simulink model "AFCSModel"  (R2025b)
settings: Solver=ode4  StartTime=0.0  StopTime=200  FixedStep=0.01  RelTol=1e-3  EnableMultiTasking=on
values from neighbouring files (symbols this model uses):
  AD = [0.05526	0.05526	0.05568	0.05804	0.06460	0.08210 ... (first row only)    [AirCraftData.m]
  Alpha0 = [0.143	0.143	0.122	-0.267	-0.627	0.120 ... (first row only)    [AirCraftData.m]
  alt = 1284.73    [Start.m]    (also in drl_simplified_dynamics.m)
  CA = 3.451    [AirCraftData.m]    (also in AircraftTrim.m)
  CDmin = [0.03799	0.03799	0.03799	0.03799	0.03904	0.04277 ... (first row only)    [AirCraftData.m]
  CLAlpha = [0.1012	0.1021	0.1033	0.1051	0.1079	0.0976 ... (first row only)    [AirCraftData.m]
  Clbt0 = [-0.00147	-0.00148	-0.00149	-0.00153	-0.00158	-0.00171 ... (first row only)    [AirCraftData.m]
  Clbtaf = [0	0	0	0	0	0;0	 0	0	0	0	0]    [AirCraftData.m]
  ClDelA = [-0.003110	-0.003065	-0.003040	-0.003036	-0.003052	-0.003088 ... (first row only)    [AirCraftData.m]
  CLDelE = [0.00653	0.00668	0.00690	0.00724	0.00772	0.00846 ... (first row only)    [AirCraftData.m]
  ClDelR = [0.000584	0.000605	0.000638	0.000686	0.000760	0.000877 ... (first row only)    [AirCraftData.m]
  CLDM = [0.244	0.244	0.244	0.244	0.244	0.244 ... (first row only)    [AirCraftData.m]
  Clp0 = [-0.5510 	-0.5610 	-0.5767 	-0.6005 	-0.6224 	-0.6763 ... (first row only)    [AirCraftData.m]
  ClpAf = [0,0,0,0,0,0;0,0,0,0,0,0]    [AirCraftData.m]
  Clr0 = [0.1308 	0.1339 	0.1383 	0.1474 	0.1601 	0.1738 ... (first row only)    [AirCraftData.m]
  ClrAf = [0,0,0,0,0,0;0,0,0,0,0,0]    [AirCraftData.m]
  Cm0 = [0.2014	0.2017	0.2034	0.2083	0.2207	0.2475 ... (first row only)    [AirCraftData.m]
  CmAfdot = [-11.5890 	-12.0169 	-12.7558 	-13.8010 	-15.2088 	-16.2278 ... (first row only)    [AirCraftData.m]
  CmCl = [-0.3454	-0.3441	-0.3427	-0.3412	-0.3396	-0.3379 ... (first row only)    [AirCraftData.m]
  CmDelE = [-0.03554	-0.03651	-0.03802	-0.04028	-0.04365	-0.04798 ... (first row only)    [AirCraftData.m]
  Cmq0 = [-42.0260 	-42.2665 	-42.9499 	-44.8315 	-45.5877 	-46.0842 ... (first row only)    [AirCraftData.m]
  CN1A0 = [0.0740	0.0662	0.0605	0.0552	0.0554 ... (first row only)    [AirCraftData.m]
  Cnbt0 = [0.00180	0.00183	0.00187	0.00192	0.00200	0.00207 ... (first row only)    [AirCraftData.m]
  Cnbtaf = [-0.000030 	-0.000031 	-0.000031 	-0.000032 	-0.000033 	-0.000035 ... (first row only)    [AirCraftData.m]
  CnDelA0 = [-0.000180	-0.000178	-0.000176	-0.000176	-0.000177	-0.000179 ... (first row only)    [AirCraftData.m]
  CnDelAAf = [0	 0	0	0	0	0;0	 0	0	0	0	0]    [AirCraftData.m]
  CnDelR = [-0.002214	-0.002274	-0.002367	-0.002505	-0.002712	-0.003039 ... (first row only)    [AirCraftData.m]
  Cnp0 = [0.0521 	0.0532 	0.0571 	0.0601 	0.0636 	0.0664 ... (first row only)    [AirCraftData.m]
  CnpAf = [0,0,0,0,0,0;0,0,0,0,0,0]    [AirCraftData.m]
  Cnr = [-0.1810 	-0.1832 	-0.1855 	-0.1892 	-0.1933 	-0.1973 ... (first row only)    [AirCraftData.m]
  Cxh_Slip = [0.0000, 0.0045, 0.0089, 0.0132, 0.0174 ... (first row only)    [AirCraftData.m]
  Cybeta0 = [-0.01783	-0.01790	-0.01804	-0.01824	-0.01851	-0.01884 ... (first row only)    [AirCraftData.m]
  Cybtaf = [0 0 0 0 0 0;0 0 0 0 0 0]    [AirCraftData.m]
  CyDelA = [0.000287	0.000295	0.000307	0.000325	0.000351	0.000394 ... (first row only)    [AirCraftData.m]
  CyDelR = [0.004946	0.005035	0.005316	0.005791	0.006458	0.007318 ... (first row only)    [AirCraftData.m]
  Cyh_Slip = [0.0000, -0.0248, -0.0519, -0.0813, -0.1130 ... (first row only)    [AirCraftData.m]
  ETA_data = [0.729 0.727 0.72 0.71 0.877 0.858 0.855 0.853 0.857 0.862 0.87 0.796 ... (330 elements, 11x5x6)]    [ETA_data.mat]
  eul_0 = [0/57.3 0/57.3 0/57.3]    [AircraftTrim.m]
  F = A(:, 1)    [drl_simplified_dynamics.m]    (also in func_DrawAircraftModel.m = [         1,  2,  3,  1;         1,  3,  4,  1;         1,  )
  flap = 0    [AircraftTrim.m]
  inertia = [  Ix      Iy     Iz  Ixz]    [AircraftTrim.m]
  Initi_Heading = 15.95*pi/180    (= 0.278380015693)    [Start.m]
  Initi_Lati = 32.6261    [Start.m]
  Initi_Longi = 103.5940    (= 103.594)    [Start.m]
  mass = 54000    [Start.m]    (also in drl_simplified_dynamics.m)
  op = evalin('base', 'op')    [drl_simplified_dynamics.m]
  q = func_GreatCircleForward(start_lat, start_lon, leg_bearing, local_s)    [system_model_update.m]
  r = r1 + r2    [drl_piecewise_reward.m]    (also in drl_reward_function.m)
  RNPAR_FlightPlan = JiuZhaiHuangLong_RNPAR_FlightPlan    [Manuscript_RNPAR_FlightPlan.m]
  Vab_0 = [Vt 0 0]    [AircraftTrim.m]
  Vt = 80    [Start.m]    (also in drl_simplified_dynamics.m; setup_afcs_system_model_test.m)
  wind_direction = 0    [Start.m]
  wind_type = 2    [Start.m]
  Wxyz_0 = [0 0 0]    [AircraftTrim.m]
  X = 1.06    [AircraftTrim.m]
  xme_0 = [0 0 -alt]    [AircraftTrim.m]
  Y = 1.177    [AircraftTrim.m]
undefined symbols (not defined in the file or in its folder): func_SystemModelMonitorBlock, Light, MIL, slselsubs, thrust_data
libraries: simulink_extras x4, aerolibatmos2 x3, aerolibconvert2 x3, aerolibwind2 x3, sharedutil x2, aerolibobsolete x1
(part 1 of 3)
settings Model: Creator=Administrator  LastModifiedBy=19894
settings SolverCC: AlgebraicLoopSolver=TrustRegion
settings DataIOCC: LimitDataPoints=on  SaveFormat=Array  SignalLoggingSaveFormat=ModelDataLogs  ReturnWorkspaceOutputs=off
settings OptimizationCC: DefaultParameterBehavior=Inlined  BufferReuse=off  ExpressionDepthLimit=2147483647.0  InitFltsAndDblsToZero=on  LifeSpan=inf
settings DebuggingCC: AlgebraicLoopMsg=none  SaveWithParameterizedLinksMsg=none  UnderspecifiedInitializationDetection=Classic  MergeDetectMultiDrivingBlocksExec=none  SignalResolutionControl=TryResolveAllWithWarning  MultiTaskDSMMsg=warning  MultiTaskCondExecSysMsg=none  FcnCallInpInsideContextMsg=warning  StateNameClashWarn=warning  SFUnexpectedBacktrackingDiag=warning  SFNoUnconditionalDefaultTransitionDiag=warning  SFExecutionAtInitializationDiag=none  ArithmeticOperatorsInVariantConditions=warning
settings HardwareCC: ProdBitPerPointer=32.0  ProdBitPerSizeT=32.0  ProdBitPerPtrDiffT=32.0  ProdLargestAtomicFloat=None  ProdIntDivRoundTo=Undefined  ProdEndianess=Unspecified  ProdWordSize=32.0  ProdHWDeviceType=32-bit Generic
settings ModelReferenceCC: PropagateSignalLabelsOutOfModel=off
settings SFSimCC: SimUseLocalCustomCode=off  CustomCodeUndefinedFunction=UseInterfaceOnly
settings RTWCC: RTWUseLocalCustomCode=off  GPUComputeCapability=3.5
settings CodeAppCC: StateflowObjectComments=on
settings GRTTargetCC: TargetFcnLib=ansi_tfl_tmw.mat  TargetLangStandard=C89/C90 (ANSI)  CombineOutputUpdateFcns=off  GRTInterface=on
settings ConfigComp: CovMetricSettings=dw  CovSaveCumulativeToWorkspaceVar=on  CovSaveSingleToWorkspaceVar=on  CovExternalEMLEnable=off  CovSFcnEnable=off

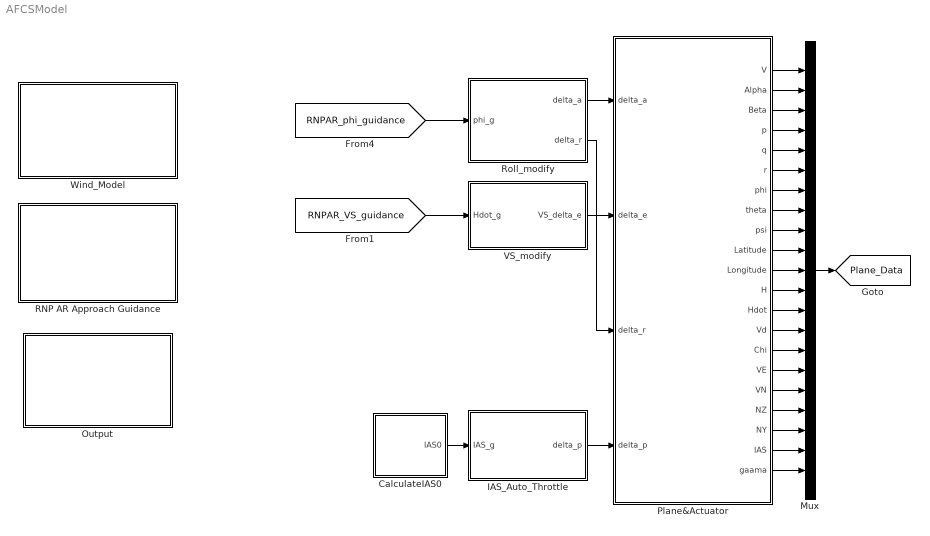
== system AFCSModel ==
  CalculateIAS0 : Subsystem
  IAS_Auto_Throttle : Subsystem
  Mux : Mux  Inputs=21
  Output : Subsystem
  Plane&Actuator : Subsystem
  RNP AR Approach Guidance : Subsystem
  Roll_modify : Subsystem
  VS_modify : Subsystem
  Wind_Model : Subsystem
  tag scope: Plane_Data=global
  wires:
  Plane&Actuator/3(Beta) -> Mux/3
  Plane&Actuator/2(Alpha) -> Mux/2
  Plane&Actuator/5(q) -> Mux/5
  Plane&Actuator/4(p) -> Mux/4
  Plane&Actuator/1(V) -> Mux/1
  Plane&Actuator/10(Latitude) -> Mux/10
  Plane&Actuator/7(phi) -> Mux/7
  Plane&Actuator/9(psi) -> Mux/9
  Plane&Actuator/12(H) -> Mux/12
  Plane&Actuator/6(r) -> Mux/6
  Plane&Actuator/11(Longitude) -> Mux/11
  Plane&Actuator/13(Hdot) -> Mux/13
  Plane&Actuator/17(VN) -> Mux/17
  Plane&Actuator/18(NZ) -> Mux/18
  Plane&Actuator/20(IAS) -> Mux/20
  Plane&Actuator/15(Chi) -> Mux/15
  Plane&Actuator/16(VE) -> Mux/16
  Plane&Actuator/19(NY) -> Mux/19
  Plane&Actuator/14(Vd) -> Mux/14
  Plane&Actuator/8(theta) -> Mux/8
  Mux/1 -> [Plane_Data]
  Plane&Actuator/21(gaama) -> Mux/21
  VS_modify/1(VS_delta_e) -> Plane&Actuator/2(delta_e)
  Roll_modify/1(delta_a) -> Plane&Actuator/1(delta_a)
  Roll_modify/2(delta_r) -> Plane&Actuator/3(delta_r)
  IAS_Auto_Throttle/1(delta_p) -> Plane&Actuator/4(delta_p)
  CalculateIAS0/1(IAS0) -> IAS_Auto_Throttle/1(IAS_g)
  [RNPAR_VS_guidance] -> VS_modify/1(Hdot_g)
  [RNPAR_phi_guidance] -> Roll_modify/1(phi_g)

== system AFCSModel/CalculateIAS0 ==
  Constant : Constant  Value=Vt
  Constant1 : Constant  Value=alt
  TAS-EAS1 : Subsystem
  IAS0 : Outport
  wires:
  Constant/1 -> TAS-EAS1/1(TAS  (m/s))
  Constant1/1 -> TAS-EAS1/2(Height  (m))
  TAS-EAS1/1(EAS (m/s)) -> IAS0/1

== system AFCSModel/IAS_Auto_Throttle ==
  IAS_g : Inport
  IAS_Controller : Subsystem
  Selector2 : Selector  InputPortWidth=21  IndexOptions=Index vector (dialog)  Indices=20  OutputSizes=1
  delta_p : Outport
  wires:
  IAS_g/1 -> IAS_Controller/1(IAS_g)
  IAS_Controller/1(delta_p) -> delta_p/1
  [Plane_Data] -> Selector2/1
  Selector2/1 -> IAS_Controller/2(IAS)

== system AFCSModel/Output ==
  note: Plane_Data  Unit:
      | V:                    m/s
      | Alpha:             rad
      | Beta:               rad
      | p:                    rad/s
      | q:                    rad/s
      | r:                     rad/s
      | phi:                 rad
      | theta:              rad
      | psi:                  rad
      | Latitude:         deg
      | Longitude:      deg
      | H:                    m
      | Hdot:               m/s
      | Vd:                  m/s
      | Chi:                 rad
      | VE:                  m/s
      | VN:                  m/s
      | NZ:                    \
      | NY:                    \
      | IAS:                 m/s
      | gaama：         rad
  Clock : Clock
  Constant : Constant  Value=110
  Gain : Gain  Gain=180/pi
  Integrator : Integrator
  Relational Operator : RelationalOperator  Operator=<=  OutDataTypeStr=boolean  InputSameDT=off
  Scope : Scope
  Scope1 : Scope
      settings: DataLoggingVariableName=ScopeData3
  Selector1 : Selector  InputPortWidth=21  IndexOptions=Index vector (dialog)  Indices=1  OutputSizes=1
  Selector2 : Selector  InputPortWidth=21  IndexOptions=Index vector (dialog)  Indices=10  OutputSizes=1
  Selector3 : Selector  InputPortWidth=21  IndexOptions=Index vector (dialog)  Indices=11  OutputSizes=1
  Selector4 : Selector  InputPortWidth=21  IndexOptions=Index vector (dialog)  Indices=12  OutputSizes=1
  Selector5 : Selector  InputPortWidth=21  IndexOptions=Index vector (dialog)  Indices=14  OutputSizes=1
  Selector6 : Selector  InputPortWidth=21  IndexOptions=Index vector (dialog)  Indices=20  OutputSizes=1
  Selector7 : Selector  InputPortWidth=21  IndexOptions=Index vector (dialog)  Indices=9  OutputSizes=1
  Stop Simulation : Stop
  To Workspace1 : ToWorkspace  VariableName=Plane_TAS  SampleTime=-1
  To Workspace2 : ToWorkspace  VariableName=Plane_Lati  SampleTime=-1
  To Workspace3 : ToWorkspace  VariableName=Plane_Longi  SampleTime=-1
  To Workspace4 : ToWorkspace  VariableName=Plane_Height  SampleTime=-1
  To Workspace5 : ToWorkspace  VariableName=Plane_Vground  SampleTime=-1
  To Workspace6 : ToWorkspace  VariableName=Plane_IAS  SampleTime=-1
  To Workspace7 : ToWorkspace  VariableName=Sim_time  SampleTime=-1
  To Workspace8 : ToWorkspace  VariableName=FlightDistance  SampleTime=-1
  wires:
  [Plane_Data] -> Selector7/1, Selector6/1, Selector5/1, Selector4/1, Selector2/1, Selector3/1, Selector1/1
  Selector1/1 -> To Workspace1/1
  Selector2/1 -> To Workspace2/1
  Selector3/1 -> To Workspace3/1
  Selector4/1 -> Relational Operator/1, Scope/1, To Workspace4/1
  Selector5/1 -> Integrator/1, To Workspace5/1
  Selector6/1 -> To Workspace6/1
  Selector7/1 -> Gain/1
  Gain/1 -> Scope1/1
  Clock/1 -> To Workspace7/1
  Relational Operator/1 -> Stop Simulation/1
  Constant/1 -> Relational Operator/2
  Integrator/1 -> To Workspace8/1

== system AFCSModel/Plane&Actuator ==
  note: Plane_Data  Unit:
      | V:                    m/s
      | Alpha:             rad
      | Beta:               rad
      | p:                    rad/s
      | q:                    rad/s
      | r:                     rad/s
      | phi:                 rad
      | theta:              rad
      | psi:                  rad
      | Latitude:         deg
      | Longitude:      deg
      | H:                    m
      | Hdot:               m/s
      | Vd:                  m/s
      | Chi:                 rad
      | VE:                  m/s
      | VN:                  m/s
      | NZ:                    \
      | NY:                    \
      | IAS:                 m/s
      | gaama：         rad
  delta_a : Inport
  delta_e : Inport  Port=2
  delta_r : Inport  Port=3
  delta_p : Inport  Port=4
  Actuator : Subsystem
  PlaneModel : Subsystem
  V : Outport
  Alpha : Outport  Port=2
  Beta : Outport  Port=3
  p : Outport  Port=4
  q : Outport  Port=5
  r : Outport  Port=6
  phi : Outport  Port=7
  theta : Outport  Port=8
  psi : Outport  Port=9
  Latitude : Outport  Port=10
  Longitude : Outport  Port=11
  H : Outport  Port=12
  Hdot : Outport  Port=13
  Vd : Outport  Port=14
  Chi : Outport  Port=15
  VE : Outport  Port=16
  VN : Outport  Port=17
  NZ : Outport  Port=18
  NY : Outport  Port=19
  IAS : Outport  Port=20
  gaama : Outport  Port=21
  wires:
  delta_a/1 -> Actuator/1(delta_a_c)
  delta_e/1 -> Actuator/2(delta_e_c)
  delta_r/1 -> Actuator/3(delta_r_c)
  delta_p/1 -> Actuator/4(delta_p_c)
  PlaneModel/1(V) -> V/1
  PlaneModel/2(Alpha) -> Alpha/1
  PlaneModel/3(Beta) -> Beta/1
  PlaneModel/4(p) -> p/1
  PlaneModel/5(q) -> q/1
  PlaneModel/6(r) -> r/1
  PlaneModel/7(phi) -> phi/1
  PlaneModel/9(psi) -> psi/1
  PlaneModel/10(Latitude) -> Latitude/1
  PlaneModel/11(Longitude) -> Longitude/1
  PlaneModel/12(H) -> H/1
  PlaneModel/13(Hdot) -> Hdot/1
  PlaneModel/14(Vd) -> Vd/1
  PlaneModel/15(Chi) -> Chi/1
  PlaneModel/16(VE) -> VE/1
  PlaneModel/17(VN) -> VN/1
  PlaneModel/18(NZ) -> NZ/1
  PlaneModel/19(NY) -> NY/1
  PlaneModel/20(IAS) -> IAS/1
  PlaneModel/21(gaama) -> gaama/1
  PlaneModel/8(theta) -> theta/1
  Actuator/1(delta_a) -> PlaneModel/1(delta_a)
  Actuator/2(delta_e) -> PlaneModel/2(delta_e)
  Actuator/3(delta_r) -> PlaneModel/3(delta_r)
  Actuator/4(delta_p) -> PlaneModel/4(delta_p)

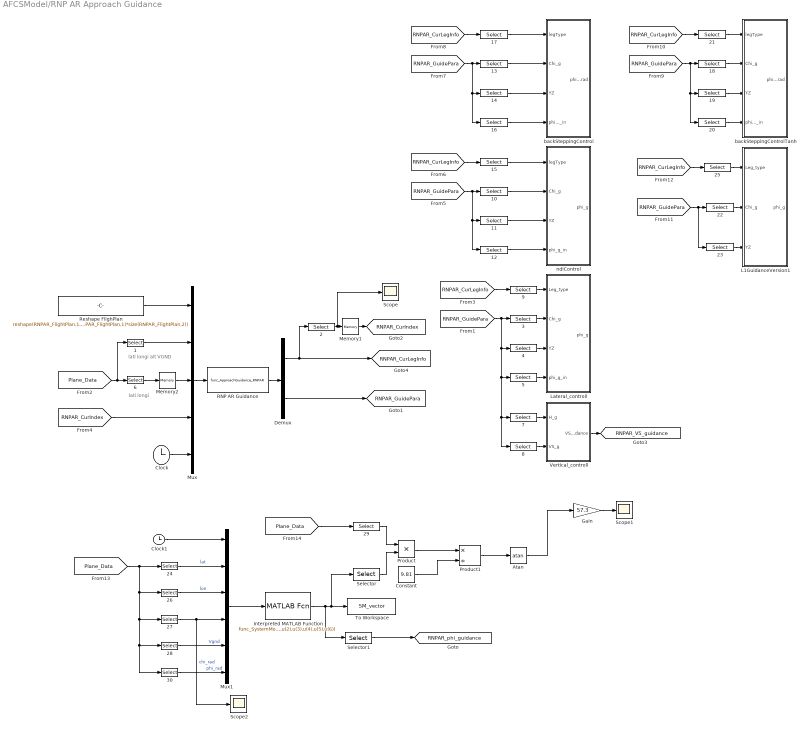
== system AFCSModel/RNP AR Approach Guidance ==
  note: lati
      | longi
  note: lati
      | longi
      | alt
      | VGND
  1 : Selector  InputPortWidth=21  IndexOptions=Index vector (dialog)  Indices=[10 11 12 14]  OutputSizes=[(-2)]
  {3,10,13,18,22} (5 alike) : Selector  InputPortWidth=5  IndexOptions=Index vector (dialog)  Indices=2  OutputSizes=[(-2)]
  {4,11,14,19,23} (5 alike) : Selector  InputPortWidth=5  IndexOptions=Index vector (dialog)  Indices=1  OutputSizes=[(-2)]
  {5,12,16,20} (4 alike) : Selector  InputPortWidth=5  IndexOptions=Index vector (dialog)  Indices=3  OutputSizes=[(-2)]
  {9,15,17,21,25} (5 alike) : Selector  InputPortWidth=16  IndexOptions=Index vector (dialog)  Indices=4  OutputSizes=[(-2)]
  2 : Selector  InputPortWidth=16  IndexOptions=Index vector (dialog)  Indices=2  OutputSizes=[(-2)]
  24 : Selector  InputPortWidth=21  IndexOptions=Index vector (dialog)  Indices=10  OutputSizes=[(-2)]
  26 : Selector  InputPortWidth=21  IndexOptions=Index vector (dialog)  Indices=11  OutputSizes=[(-2)]
  27 : Selector  InputPortWidth=21  IndexOptions=Index vector (dialog)  Indices=15  OutputSizes=[(-2)]
  28 : Selector  InputPortWidth=21  IndexOptions=Index vector (dialog)  Indices=14  OutputSizes=[(-2)]
  29 : Selector  InputPortWidth=21  IndexOptions=Index vector (dialog)  Indices=14  OutputSizes=[(-2)]
  30 : Selector  InputPortWidth=21  IndexOptions=Index vector (dialog)  Indices=7  OutputSizes=[(-2)]
  6 : Selector  InputPortWidth=21  IndexOptions=Index vector (dialog)  Indices=[10 11]  OutputSizes=[(-2)]
  7 : Selector  InputPortWidth=5  IndexOptions=Index vector (dialog)  Indices=4  OutputSizes=[(-2)]
  8 : Selector  InputPortWidth=5  IndexOptions=Index vector (dialog)  Indices=5  OutputSizes=[(-2)]
  Atan : Trigonometry  Operator=atan
  Clock : Clock
  Clock1 : Clock
  Constant : Constant  Value=9.81
  Demux : Demux  Outputs=[16 5]
  Gain : Gain  Gain=57.3
  Interpreted MATLAB Function : MATLABFcn  MATLABFcn=func_SystemModelMonitorBlock(u(1),u(2),u(3),u(4),u(5),u(6))  OutputDimensions=14
  L1GuidanceVersion1 : Subsystem
  Lateral_controll : Subsystem
  Memory1 : Memory  InitialCondition=1
  Memory2 : Memory  InitialCondition=1
  Mux : Mux  Inputs=5
  Mux1 : Mux  Inputs=6
  Product : Product
  Product1 : Product  Inputs=*/
  RNP AR Guidance : MATLABFcn  MATLABFcn=func_ApproachGuidance_RNPAR  OutputDimensions=21
  Reshape FlighPlan : Constant  Value=reshape(RNPAR_FlightPlan,1,size(RNPAR_FlightPlan,1)*size(RNPAR_FlightPlan,2))
  Scope : Scope
      settings: ActiveDisplayYMinimum=-1  ActiveDisplayYMaximum=1  DataLoggingVariableName=ScopeData2
  Scope1 : Scope
      settings: ActiveDisplayYMinimum=-1  ActiveDisplayYMaximum=1  DataLoggingVariableName=ScopeData14
  Scope2 : Scope
      settings: ActiveDisplayYMinimum=-1  ActiveDisplayYMaximum=1  DataLoggingVariableName=ScopeData15
  Selector : Selector  InputPortWidth=14  IndexOptions=Index vector (dialog)  Indices=11  OutputSizes=1
  Selector1 : Selector  InputPortWidth=14  IndexOptions=Index vector (dialog)  Indices=12  OutputSizes=1
  To Workspace : ToWorkspace  VariableName=SM_vector  SaveFormat=Timeseries  SampleTime=-1
  Vertical_controll : Subsystem
  backSteppingControl : Subsystem
  backSteppingControlTanh : Subsystem
  ndiControl : Subsystem
  tag scope: RNPAR_CurIndex=global, RNPAR_CurLegInfo=global, RNPAR_GuidePara=global, RNPAR_VS_guidance=global, RNPAR_phi_guidance=global
  wires:
  Mux/1 -> RNP AR Guidance/1
  RNP AR Guidance/1 -> Demux/1
  Demux/1 -> 2/1, [RNPAR_CurLegInfo]
  Demux/2 -> [RNPAR_GuidePara]
  Clock/1 -> Mux/5
  [RNPAR_CurIndex] -> Mux/4
  [Plane_Data] -> 1/1, 6/1
  Memory1/1 -> [RNPAR_CurIndex]
  6/1 -> Memory2/1
  Memory2/1 -> Mux/3
  1/1 -> Mux/2
  Reshape FlighPlan/1 -> Mux/1
  [RNPAR_GuidePara] -> 8/1, 7/1, 5/1, 4/1, 3/1
  7/1 -> Vertical_controll/1(H_g)
  8/1 -> Vertical_controll/2(VS_g)
  [RNPAR_CurLegInfo] -> 9/1
  [RNPAR_CurLegInfo] -> 15/1
  [RNPAR_GuidePara] -> 12/1, 11/1, 10/1
  15/1 -> ndiControl/1(legType)
  10/1 -> ndiControl/2(Chi_g)
  11/1 -> ndiControl/3(YZ)
  12/1 -> ndiControl/4(phi_g_in)
  9/1 -> Lateral_controll/1(Leg_type)
  3/1 -> Lateral_controll/2(Chi_g)
  4/1 -> Lateral_controll/3(YZ)
  5/1 -> Lateral_controll/4(phi_g_in)
  17/1 -> backSteppingControl/1(legType)
  16/1 -> backSteppingControl/4(phi_g_in)
  [RNPAR_GuidePara] -> 16/1, 14/1, 13/1
  14/1 -> backSteppingControl/3(YZ)
  [RNPAR_CurLegInfo] -> 17/1
  13/1 -> backSteppingControl/2(Chi_g)
  2/1 -> Scope/1, Memory1/1
  20/1 -> backSteppingControlTanh/4(phi_g_in)
  19/1 -> backSteppingControlTanh/3(YZ)
  [RNPAR_GuidePara] -> 20/1, 19/1, 18/1
  [RNPAR_CurLegInfo] -> 21/1
  18/1 -> backSteppingControlTanh/2(Chi_g)
  21/1 -> backSteppingControlTanh/1(legType)
  [RNPAR_GuidePara] -> 23/1, 22/1
  23/1 -> L1GuidanceVersion1/3(YZ)
  [RNPAR_CurLegInfo] -> 25/1
  22/1 -> L1GuidanceVersion1/2(Chi_g)
  25/1 -> L1GuidanceVersion1/1(Leg_type)
  Clock1/1 -> Mux1/1
  24/1 -> Mux1/2  "lat"
  26/1 -> Mux1/3  "lon"
  27/1 -> Scope2/1, Mux1/4  "chi_rad"
  28/1 -> Mux1/5  "Vgnd"
  [Plane_Data] -> 30/1, 28/1, 27/1, 26/1, 24/1
  Mux1/1 -> Interpreted MATLAB Function/1
  Interpreted MATLAB Function/1 -> Selector1/1, Selector/1, To Workspace/1
  [Plane_Data] -> 29/1
  29/1 -> Product/1
  Selector/1 -> Product/2
  Product/1 -> Product1/1
  Constant/1 -> Product1/2
  Product1/1 -> Atan/1
  Atan/1 -> Gain/1
  Gain/1 -> Scope1/1
  Vertical_controll/1(VS_Guidance) -> [RNPAR_VS_guidance]
  30/1 -> Mux1/6  "phi_rad"
  Selector1/1 -> [RNPAR_phi_guidance]

== system AFCSModel/Roll_modify ==
  note: p
  note: phi
  phi_g : Inport
  1 : Selector  InputPortWidth=21  IndexOptions=Index vector (dialog)  Indices=6  OutputSizes=[(-2)]
  5 : Selector  InputPortWidth=21  IndexOptions=Index vector (dialog)  Indices=7  OutputSizes=[(-2)]
  6 : Selector  InputPortWidth=21  IndexOptions=Index vector (dialog)  Indices=4  OutputSizes=[(-2)]
  Gain : Gain
  Gain1 : Gain
  Gain3 : Gain  Gain=-0.03
  Gain4 : Gain  Gain=-0.019
  Saturation1 : Saturate  UpperLimit=30*pi/180  LowerLimit=-30*pi/180
  Sum1 : Sum  Inputs=|++
  Sum2 : Sum
  Sum3 : Sum  Inputs=|-+
  delta_a : Outport
  delta_r : Outport  Port=2
  wires:
  Sum1/1 -> delta_a/1
  Gain3/1 -> Sum2/2
  Gain4/1 -> Sum2/1
  Sum2/1 -> delta_r/1
  Sum3/1 -> Gain/1
  Gain/1 -> Sum1/1
  Saturation1/1 -> Gain4/1, Sum3/2
  [Plane_Data] -> 1/1, 6/1, 5/1
  1/1 -> Gain3/1  "r"
  6/1 -> Gain1/1
  phi_g/1 -> Sum3/1
  5/1 -> Saturation1/1
  Gain1/1 -> Sum1/2

== system AFCSModel/VS_modify ==
  note: Hdot
  Hdot_g : Inport
  Gain1 : Gain  Gain=0.5
  Gain2 : Gain  Gain=0.2
  Gain3 : Gain  Gain=-1/57.3
  Integrator : Integrator
  Pitch_modify : Subsystem
  Saturation1 : Saturate  UpperLimit=10  LowerLimit=-10
  Selector1 : Selector  InputPortWidth=21  IndexOptions=Index vector (dialog)  Indices=13  OutputSizes=1
  Sum1 : Sum  Inputs=|++
  Sum3 : Sum  Inputs=|-+
  VS_delta_e : Outport
  wires:
  Integrator/1 -> Gain2/1
  Sum1/1 -> Gain3/1
  Gain1/1 -> Sum1/1
  Gain2/1 -> Sum1/2
  Sum3/1 -> Saturation1/1
  Saturation1/1 -> Integrator/1, Gain1/1
  Gain3/1 -> Pitch_modify/1(theta_g)
  Hdot_g/1 -> Sum3/1
  [Plane_Data] -> Selector1/1
  Selector1/1 -> Sum3/2
  Pitch_modify/1(delta_e) -> VS_delta_e/1

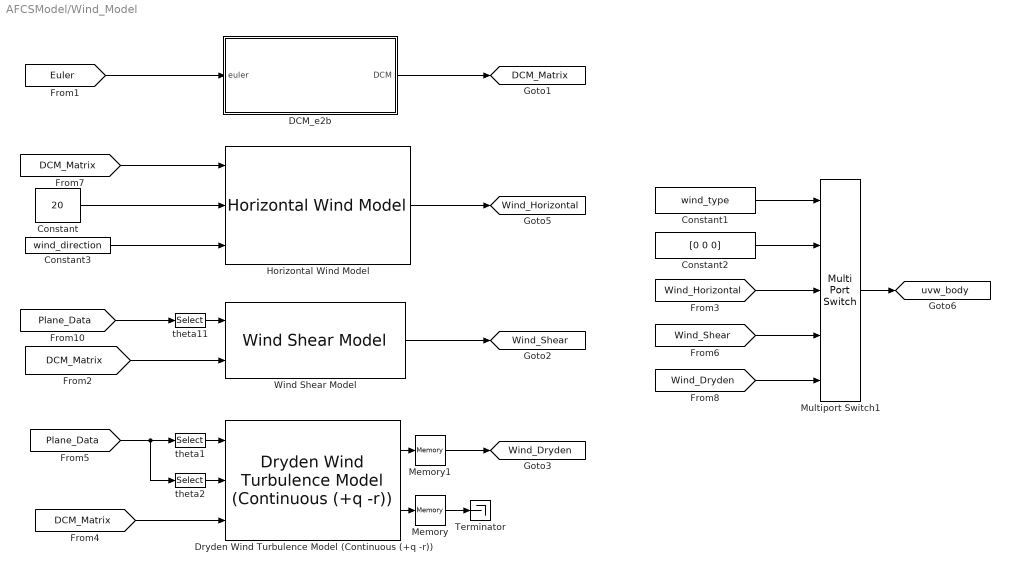
== system AFCSModel/Wind_Model ==
  Constant : Constant  Value=20
  Constant1 : Constant  Value=wind_type
  Constant2 : Constant  Value=[0 0 0]
  Constant3 : Constant  Value=wind_direction
  DCM_e2b : Subsystem
  Dryden Wind Turbulence Model (Continuous (+q -r)) : aerolibwind2/Dryden Wind Turbulence Model  (Continuous (+q -r))  units=Metric (MKS)  spec=MIL-F-8785C  model=Continuous Dryden (+q -r)  W20=2  Wdeg=0  TurbProb=10^-2 - Light  L_high=533.4  Wingspan=4  ts=0.01  Seed=[23341 23342 23343 23344]  T_on=on
  Horizontal Wind Model : aerolibwind2/Horizontal Wind Model  units=Metric (MKS)  Vw_source=External  Vwind=10  W_source=External  Wdeg=290
  Memory : Memory
  Memory1 : Memory
  Multiport Switch1 : MultiPortSwitch  Inputs=4  SaturateOnIntegerOverflow=off  InputSameDT=off
  Terminator : Terminator
  Wind Shear Model : aerolibwind2/Wind Shear Model  units=Metric (MKS)  phase=Category C - Terminal Flight Phase  W_20=1  Wdeg=0
  theta1 : Selector  InputPortWidth=21  IndexOptions=Index vector (dialog)  Indices=12  OutputSizes=[(-2)]
  theta11 : Selector  InputPortWidth=21  IndexOptions=Index vector (dialog)  Indices=12  OutputSizes=[(-2)]
  theta2 : Selector  InputPortWidth=21  IndexOptions=Index vector (dialog)  Indices=1  OutputSizes=[(-2)]
  tag scope: DCM_Matrix=global, Wind_Dryden=global, Wind_Horizontal=global, Wind_Shear=global, uvw_body=global
  wires:
  [Euler] -> DCM_e2b/1(euler)
  DCM_e2b/1(DCM) -> [DCM_Matrix]
  [DCM_Matrix] -> Wind Shear Model/2
  theta11/1 -> Wind Shear Model/1
  [Plane_Data] -> theta2/1, theta1/1
  [DCM_Matrix] -> Dryden Wind Turbulence Model (Continuous (+q -r))/3
  theta1/1 -> Dryden Wind Turbulence Model (Continuous (+q -r))/1
  theta2/1 -> Dryden Wind Turbulence Model (Continuous (+q -r))/2
  Dryden Wind Turbulence Model (Continuous (+q -r))/1 -> Memory1/1
  [DCM_Matrix] -> Horizontal Wind Model/1
  [Plane_Data] -> theta11/1
  Dryden Wind Turbulence Model (Continuous (+q -r))/2 -> Memory/1
  Memory/1 -> Terminator/1
  Horizontal Wind Model/1 -> [Wind_Horizontal]
  Memory1/1 -> [Wind_Dryden]
  Constant/1 -> Horizontal Wind Model/2
  Constant3/1 -> Horizontal Wind Model/3
  Wind Shear Model/1 -> [Wind_Shear]
  Constant1/1 -> Multiport Switch1/1
  Multiport Switch1/1 -> [uvw_body]
  Constant2/1 -> Multiport Switch1/2
  [Wind_Horizontal] -> Multiport Switch1/3
  [Wind_Shear] -> Multiport Switch1/4
  [Wind_Dryden] -> Multiport Switch1/5

== system AFCSModel/CalculateIAS0/TAS-EAS1 ==
  TAS  (m/s) : Inport
  Height  (m) : Inport  Port=2
  Display1 : Display
  Divide : Product  Inputs=*/
  Fcn : Fcn  Expr=sqrt(u)
  ISA Atmosphere Model2 : aerolibatmos2/ISA Atmosphere Model  useExtended=off  action=Warning  custom=off  viscosityOut=off  g=9.80665  gamma=1.4  R=287.0531  L=0.0065  h_trop=11000  h_strat=20000  rho0=1.225  P0=101325  T0=288.15  h0=0  S=110.4  Tref=273.15  muref=1.716e-5
  Product : Product  RndMeth=Zero
  Rou_o : Constant  Value=1.225
  Terminator : Terminator
  Terminator1 : Terminator
  Terminator2 : Terminator
  EAS (m/s) : Outport
  wires:
  TAS  (m/s)/1 -> Product/2
  Fcn/1 -> Product/1
  ISA Atmosphere Model2/3 -> Terminator2/1
  ISA Atmosphere Model2/2 -> Terminator1/1
  ISA Atmosphere Model2/1 -> Terminator/1
  Product/1 -> EAS (m/s)/1, Display1/1
  Divide/1 -> Fcn/1
  ISA Atmosphere Model2/4 -> Divide/1
  Height  (m)/1 -> ISA Atmosphere Model2/1
  Rou_o/1 -> Divide/2

== system AFCSModel/IAS_Auto_Throttle/IAS_Controller ==
  IAS_g : Inport
  IAS : Inport  Port=2
  Gain : Gain  Gain=1.1
  Gain1 : Gain  Gain=0.0025
  Integrator : Integrator
  Sum1 : Sum  Inputs=|++
  Sum3 : Sum  Inputs=|+-
  delta_p : Outport
  wires:
  IAS/1 -> Sum3/2
  IAS_g/1 -> Sum3/1
  Sum3/1 -> Integrator/1, Gain/1
  Gain/1 -> Sum1/1
  Sum1/1 -> delta_p/1
  Integrator/1 -> Gain1/1
  Gain1/1 -> Sum1/2

== system AFCSModel/Plane&Actuator/Actuator ==
  delta_a_c : Inport
  delta_e_c : Inport  Port=2
  delta_r_c : Inport  Port=3
  delta_p_c : Inport  Port=4
  Gain1 : Gain  SaturateOnIntegerOverflow=on  OutDataTypeStr=Inherit: Same as input  ParamDataTypeStr=Inherit: Same as input
  Gain2 : Gain  Gain=1/57.3  SaturateOnIntegerOverflow=on  OutDataTypeStr=Inherit: Same as input  ParamDataTypeStr=Inherit: Same as input
  Gain3 : Gain  Gain=1/57.3  SaturateOnIntegerOverflow=on  OutDataTypeStr=Inherit: Same as input  ParamDataTypeStr=Inherit: Same as input
  Gain4 : Gain  Gain=1/57.3  SaturateOnIntegerOverflow=on  OutDataTypeStr=Inherit: Same as input  ParamDataTypeStr=Inherit: Same as input
  Gain5 : Gain  Gain=57.3  SaturateOnIntegerOverflow=on  OutDataTypeStr=Inherit: Same as input  ParamDataTypeStr=Inherit: Same as input
  Gain6 : Gain  Gain=57.3  SaturateOnIntegerOverflow=on  OutDataTypeStr=Inherit: Same as input  ParamDataTypeStr=Inherit: Same as input
  Gain7 : Gain  Gain=57.3  SaturateOnIntegerOverflow=on  OutDataTypeStr=Inherit: Same as input  ParamDataTypeStr=Inherit: Same as input
  Gain8 : Gain  Gain=3.5  SaturateOnIntegerOverflow=on  OutDataTypeStr=Inherit: Same as input  ParamDataTypeStr=Inherit: Same as input
  Gain9 : Gain  SaturateOnIntegerOverflow=on  OutDataTypeStr=Inherit: Same as input  ParamDataTypeStr=Inherit: Same as input
  actuator1 : Subsystem
  actuator3 : Subsystem
  actuator5 : Subsystem
  delta_a : Outport
  delta_e : Outport  Port=2
  delta_r : Outport  Port=3
  delta_p : Outport  Port=4
  wires:
  Gain5/1 -> Gain1/1
  delta_a_c/1 -> Gain5/1
  delta_e_c/1 -> Gain6/1
  delta_r_c/1 -> Gain7/1
  Gain1/1 -> actuator5/1(In)
  Gain8/1 -> actuator1/1(In)
  Gain9/1 -> actuator3/1(In)
  Gain3/1 -> delta_e/1
  Gain4/1 -> delta_r/1
  Gain6/1 -> Gain8/1
  Gain7/1 -> Gain9/1
  delta_p_c/1 -> delta_p/1
  actuator5/1(Out) -> Gain2/1
  actuator1/1(Out) -> Gain3/1
  actuator3/1(Out) -> Gain4/1
  Gain2/1 -> delta_a/1

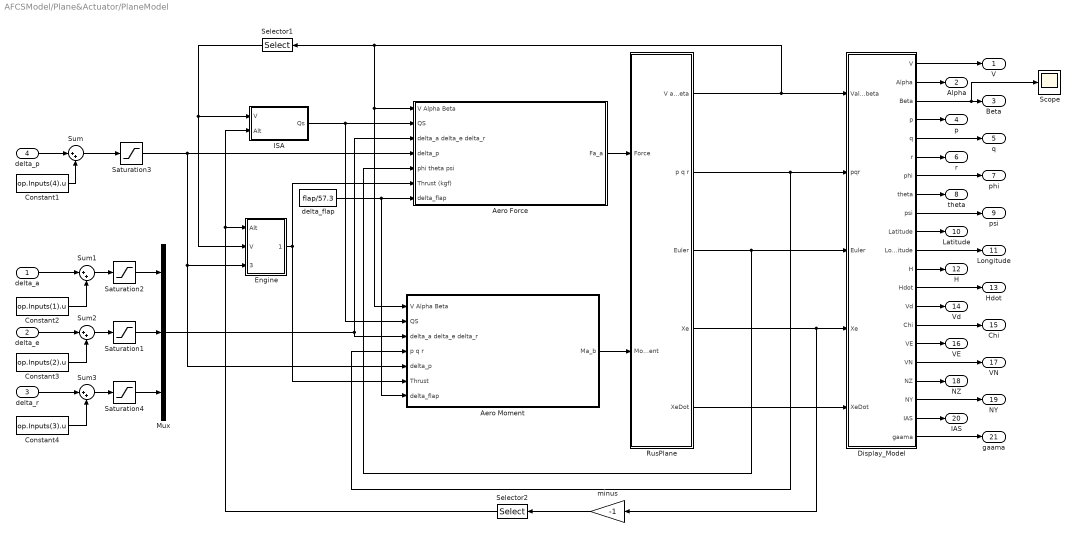
== system AFCSModel/Plane&Actuator/PlaneModel ==
  delta_a : Inport
  delta_e : Inport  Port=2
  delta_r : Inport  Port=3
  delta_p : Inport  Port=4
  Aero Force : Subsystem
  Aero Moment : Subsystem
  Constant1 : Constant  Value=op.Inputs(4).u  OutDataTypeStr=Inherit: Inherit via back propagation
  Constant2 : Constant  Value=op.Inputs(1).u  OutDataTypeStr=Inherit: Inherit via back propagation
  Constant3 : Constant  Value=op.Inputs(2).u  OutDataTypeStr=Inherit: Inherit via back propagation
  Constant4 : Constant  Value=op.Inputs(3).u  OutDataTypeStr=Inherit: Inherit via back propagation
  Display_Model : Subsystem
  Engine : Subsystem
  ISA : Subsystem
  Mux : Mux  Inputs=3
  RusPlane : Subsystem  mask{Xme_0=xme_0, Vab_0=Vab_0, eul_0=eul_0, Wxyz_0=Wxyz_0, inertia=inertia, mass=mass}
      mask prompts: Xme_0 "Initial position in inertial axes[Xe,Ye,Ze]"; Vab_0 "Initial velocity in body axes"; eul_0 "Initial Euler orientation"; Wxyz_0 "Initial body rotation rates"
  Saturation1 : Saturate  UpperLimit=21*pi/180  LowerLimit=-21*pi/180
  Saturation2 : Saturate  UpperLimit=24*pi/180  LowerLimit=-24*pi/180
  Saturation3 : Saturate  UpperLimit=1.04  LowerLimit=0
  Saturation4 : Saturate  UpperLimit=25*pi/180  LowerLimit=-25*pi/180
  Scope : Scope
      settings: ActiveDisplayYMinimum=-0.02888  ActiveDisplayYMaximum=0.01693  DataLoggingVariableName=ScopeData4
  Selector1 : Selector  InputPortWidth=3  IndexOptions=Index vector (dialog)  Indices=[1]  OutputSizes=[(-2)]
  Selector2 : Selector  InputPortWidth=3  IndexOptions=Index vector (dialog)  Indices=[3]  OutputSizes=[(-2)]
  Sum{,1..3} (4 alike) : Sum  Inputs=|++
  delta_flap : Constant  Value=flap/57.3
  minus : Gain  Gain=-1
  V : Outport
  Alpha : Outport  Port=2
  Beta : Outport  Port=3
  p : Outport  Port=4
  q : Outport  Port=5
  r : Outport  Port=6
  phi : Outport  Port=7
  theta : Outport  Port=8
  psi : Outport  Port=9
  Latitude : Outport  Port=10
  Longitude : Outport  Port=11
  H : Outport  Port=12
  Hdot : Outport  Port=13
  Vd : Outport  Port=14
  Chi : Outport  Port=15
  VE : Outport  Port=16
  VN : Outport  Port=17
  NZ : Outport  Port=18
  NY : Outport  Port=19
  IAS : Outport  Port=20
  gaama : Outport  Port=21
  wires:
  Aero Force/1(Fa_a) -> RusPlane/1(Force)
  minus/1 -> Selector2/1
  RusPlane/1(V alpha beta) -> Aero Moment/1(V Alpha Beta), Aero Force/1(V Alpha Beta), Selector1/1, Display_Model/1(Valphabeta)
  RusPlane/2(p q r) -> Aero Moment/4(p q r), Display_Model/2(pqr)
  RusPlane/3(Euler) -> Aero Force/5(phi theta psi), Display_Model/3(Euler)
  RusPlane/4(Xe) -> minus/1, Display_Model/4(Xe)
  Selector1/1 -> Engine/2(V), ISA/1(V)
  ISA/1(Qs) -> Aero Moment/2(QS), Aero Force/2(QS)
  Engine/1(Thrust) -> Aero Force/6(Thrust (kgf)), Aero Moment/6(Thrust)
  Selector2/1 -> ISA/2(Alt), Engine/1(Alt)
  Mux/1 -> Aero Force/3(delta_a delta_e delta_r), Aero Moment/3(delta_a delta_e delta_r)
  Sum/1 -> Saturation3/1
  delta_flap/1 -> Aero Moment/7(delta_flap), Aero Force/7(delta_flap)
  Constant1/1 -> Sum/2
  delta_p/1 -> Sum/1
  delta_a/1 -> Sum1/1
  Sum1/1 -> Saturation2/1
  Constant2/1 -> Sum1/2
  delta_e/1 -> Sum2/1
  Sum2/1 -> Saturation1/1
  Constant3/1 -> Sum2/2
  delta_r/1 -> Sum3/1
  Sum3/1 -> Saturation4/1
  Constant4/1 -> Sum3/2
  Aero Moment/1(Ma_b) -> RusPlane/2(Moment)
  RusPlane/5(XeDot) -> Display_Model/5(XeDot)
  Display_Model/1(V) -> V/1
  Display_Model/2(Alpha) -> Alpha/1
  Display_Model/3(Beta) -> Scope/1, Beta/1
  Saturation3/1 -> Aero Moment/5(delta_p), Engine/3(delta_p), Aero Force/4(delta_p)
  Saturation1/1 -> Mux/2
  Saturation2/1 -> Mux/1
  Saturation4/1 -> Mux/3
  Display_Model/4(p) -> p/1
  Display_Model/5(q) -> q/1
  Display_Model/6(r) -> r/1
  Display_Model/7(phi) -> phi/1
  Display_Model/8(theta) -> theta/1
  Display_Model/9(psi) -> psi/1
  Display_Model/10(Latitude) -> Latitude/1
  Display_Model/11(Longitude) -> Longitude/1
  Display_Model/12(H) -> H/1
  Display_Model/13(Hdot) -> Hdot/1
  Display_Model/14(Vd) -> Vd/1
  Display_Model/15(Chi) -> Chi/1
  Display_Model/16(VE) -> VE/1
  Display_Model/17(VN) -> VN/1
  Display_Model/18(NZ) -> NZ/1
  Display_Model/19(NY) -> NY/1
  Display_Model/20(IAS) -> IAS/1
  Display_Model/21(gaama) -> gaama/1

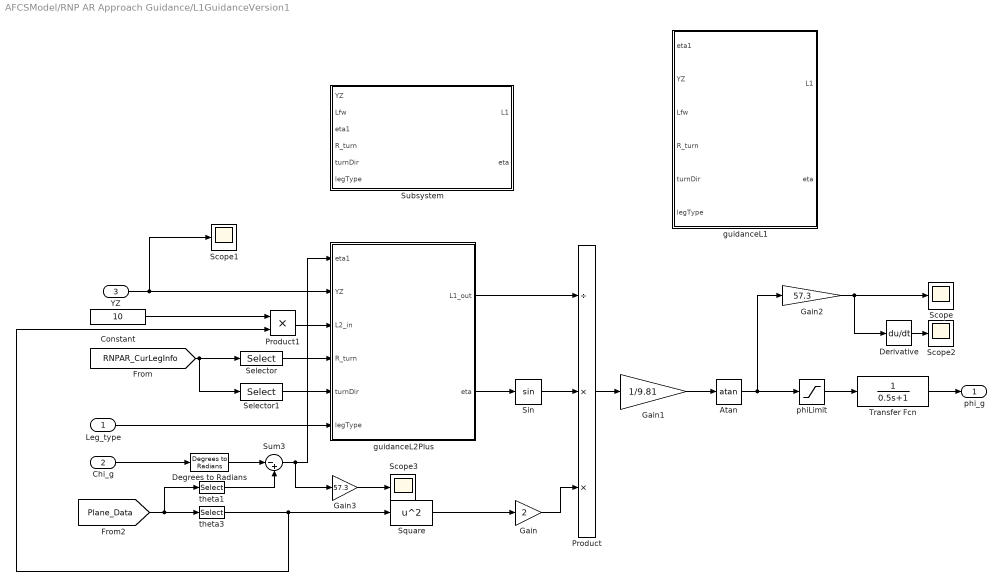
== system AFCSModel/RNP AR Approach Guidance/L1GuidanceVersion1 ==
  Leg_type : Inport
  Chi_g : Inport  Port=2
  YZ : Inport  Port=3
  Atan : Trigonometry  Operator=atan
  Constant : Constant  Value=10
  Degrees to Radians : simulink_extras/Transformations/Degrees to Radians
  Derivative : Derivative
  Gain : Gain  Gain=2
  Gain1 : Gain  Gain=1/9.81
  Gain2 : Gain  Gain=57.3
  Gain3 : Gain  Gain=57.3
  Product : Product  Inputs=/**
  Product1 : Product
  Scope{,1..3} (4 alike) : Scope
      Scope settings: ActiveDisplayYMinimum=-49.700338385944981  ActiveDisplayYMaximum=69.674230856158971  DataLoggingVariableName=ScopeData7
      Scope1 settings: ActiveDisplayYMinimum=-263.74531992815992  ActiveDisplayYMaximum=1408.7169624432363  DataLoggingVariableName=ScopeData11
      Scope2 settings: ActiveDisplayYMinimum=-2627.3493181445187  ActiveDisplayYMaximum=5118.8487000051327  DataLoggingVariableName=ScopeData12
      Scope3 settings: ActiveDisplayYMinimum=-15.030226123152808  ActiveDisplayYMaximum=57.345652596596693  DataLoggingVariableName=ScopeData13
  Selector : Selector  InputPortWidth=16  IndexOptions=Index vector (dialog)  Indices=16  OutputSizes=1
  Selector1 : Selector  InputPortWidth=16  IndexOptions=Index vector (dialog)  Indices=15  OutputSizes=1
  Sin : Trigonometry
  Square : Math  Operator=square
  Subsystem : Subsystem
  Sum3 : Sum  Inputs=|-+
  Transfer Fcn : TransferFcn  Denominator=[0.5 1]
  guidanceL1 : MATLAB Function  TreatAsAtomicUnit=on
  guidanceL2Plus : MATLAB Function  TreatAsAtomicUnit=on
  phiLimit : Saturate  UpperLimit=30/57.3  LowerLimit=-30/57.3
  theta1 : Selector  InputPortWidth=21  IndexOptions=Index vector (dialog)  Indices=15  OutputSizes=[(-2)]
  theta3 : Selector  InputPortWidth=21  IndexOptions=Index vector (dialog)  Indices=14  OutputSizes=[(-2)]
  phi_g : Outport
  wires:
  Chi_g/1 -> Degrees to Radians/1
  [Plane_Data] -> theta3/1, theta1/1
  Degrees to Radians/1 -> Sum3/1
  theta3/1 -> Square/1, Product1/2
  Square/1 -> Gain/1
  Sin/1 -> Product/2
  Gain/1 -> Product/3
  Product/1 -> Gain1/1
  Gain1/1 -> Atan/1
  Atan/1 -> Gain2/1, phiLimit/1
  Gain2/1 -> Scope/1, Derivative/1
  phiLimit/1 -> Transfer Fcn/1
  Derivative/1 -> Scope2/1
  [RNPAR_CurLegInfo] -> Selector1/1, Selector/1
  guidanceL2Plus/2(eta) -> Sin/1
  Selector/1 -> guidanceL2Plus/4(R_turn)
  Selector1/1 -> guidanceL2Plus/5(turnDir)
  Leg_type/1 -> guidanceL2Plus/6(legType)
  Sum3/1 -> Gain3/1, guidanceL2Plus/1(eta1)
  YZ/1 -> Scope1/1, guidanceL2Plus/2(YZ)
  Transfer Fcn/1 -> phi_g/1
  theta1/1 -> Sum3/2
  Product1/1 -> guidanceL2Plus/3(L2_in)
  Constant/1 -> Product1/1
  guidanceL2Plus/1(L1_out) -> Product/1
  Gain3/1 -> Scope3/1

== system AFCSModel/RNP AR Approach Guidance/Lateral_controll ==
  Leg_type : Inport
  Chi_g : Inport  Port=2
  YZ : Inport  Port=3
  phi_g_in : Inport  Port=4
  30 : Saturate  UpperLimit=30  LowerLimit=-30
  Angle Conversion2 : aerolibconvert2/Angle Conversion  IU=rad  OU=deg
  Derivative : Derivative
  Gain : Gain  Gain=pi/180
  Gain1 : Gain  Gain=0.2
  Gain2 : Gain  Gain=3
  Gain4 : Gain  Gain=0.3
  Gain5 : Gain  Gain=-0.03
  Product : Product
  Scope : Scope
      settings: ActiveDisplayYMinimum=-765.873933362086  ActiveDisplayYMaximum=94.341204978904187
  Sum2 : Sum  Inputs=|++
  Sum3 : Sum  Inputs=|-+
  Sum4 : Sum  Inputs=+++
  Switch : Switch  Criteria=u2 > Threshold  Threshold=0.5  SaturateOnIntegerOverflow=off  InputSameDT=off
  theta1 : Selector  InputPortWidth=21  IndexOptions=Index vector (dialog)  Indices=15  OutputSizes=[(-2)]
  theta3 : Selector  InputPortWidth=21  IndexOptions=Index vector (dialog)  Indices=14  OutputSizes=[(-2)]
  phi_g : Outport
  wires:
  Leg_type/1 -> Switch/2
  Chi_g/1 -> Sum3/1
  theta3/1 -> Product/2
  Product/1 -> Gain5/1
  Sum2/1 -> Switch/3
  phi_g_in/1 -> Sum4/1
  Sum4/1 -> Switch/1
  Switch/1 -> 30/1
  YZ/1 -> Scope/1, Gain1/1, Derivative/1, Gain4/1
  30/1 -> Gain/1
  Gain1/1 -> Sum2/1
  Gain5/1 -> Sum2/2
  [Plane_Data] -> theta3/1, theta1/1
  theta1/1 -> Angle Conversion2/1
  Gain/1 -> phi_g/1
  Sum3/1 -> Product/1
  Gain4/1 -> Sum4/2
  Derivative/1 -> Gain2/1
  Gain2/1 -> Sum4/3
  Angle Conversion2/1 -> Sum3/2

== system AFCSModel/RNP AR Approach Guidance/Vertical_controll ==
  H_g : Inport
  VS_g : Inport  Port=2
  10 : Saturate  UpperLimit=10  LowerLimit=-10
  Gain3 : Gain
  Gain4 : Gain  Gain=0.1
  Sum1 : Sum  Inputs=|+-
  Sum4 : Sum  Inputs=++|
  theta3 : Selector  InputPortWidth=21  IndexOptions=Index vector (dialog)  Indices=12  OutputSizes=[(-2)]
  VS_Guidance : Outport
  wires:
  10/1 -> VS_Guidance/1
  VS_g/1 -> Gain3/1
  Gain4/1 -> Sum4/2
  Gain3/1 -> Sum4/1
  H_g/1 -> Sum1/1
  theta3/1 -> Sum1/2
  [Plane_Data] -> theta3/1
  Sum1/1 -> Gain4/1
  Sum4/1 -> 10/1

== system AFCSModel/RNP AR Approach Guidance/backSteppingControl ==
  note: 反步控制
  legType : Inport
  Chi_g : Inport  Port=2
  YZ : Inport  Port=3
  phi_g_in : Inport  Port=4
  Degrees to Radians : simulink_extras/Transformations/Degrees to Radians
  Scope : Scope
      settings: ActiveDisplayYMinimum=-33.423150826962029  ActiveDisplayYMaximum=28.813687017181081
  Scope2 : Scope
      settings: ActiveDisplayYMinimum=-0.2622  ActiveDisplayYMaximum=0.24597  DataLoggingVariableName=ScopeData6
  caculatePhi : Subsystem
  deltaChi : Sum  Inputs=-+|
  g : Constant  Value=9.81
  k1 : Constant  Value=0.02
  k2 : Constant  Value=0.3
  phiLimit : Saturate  UpperLimit=30/57.3  LowerLimit=-30/57.3
  theta1 : Selector  InputPortWidth=21  IndexOptions=Index vector (dialog)  Indices=15  OutputSizes=[(-2)]
  theta3 : Selector  InputPortWidth=21  IndexOptions=Index vector (dialog)  Indices=14  OutputSizes=[(-2)]
  phi_g_rad : Outport
  wires:
  [Plane_Data] -> theta3/1, theta1/1
  phiLimit/1 -> Scope2/1, phi_g_rad/1
  Chi_g/1 -> Degrees to Radians/1
  theta1/1 -> deltaChi/2
  Degrees to Radians/1 -> deltaChi/1
  YZ/1 -> Scope/1, caculatePhi/1(YZ)
  k1/1 -> caculatePhi/2(k1)
  k2/1 -> caculatePhi/3(k2)
  deltaChi/1 -> caculatePhi/4(deltaChi)
  theta3/1 -> caculatePhi/5(vGnd)
  g/1 -> caculatePhi/6(g)
  caculatePhi/1(phiControl) -> phiLimit/1
  legType/1 -> caculatePhi/7(legType)
  phi_g_in/1 -> caculatePhi/8(phi_g_in)

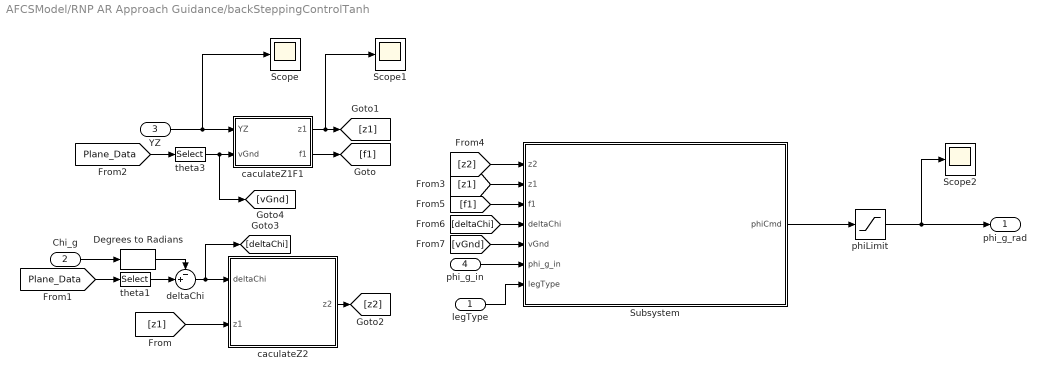
== system AFCSModel/RNP AR Approach Guidance/backSteppingControlTanh ==
  legType : Inport
  Chi_g : Inport  Port=2
  YZ : Inport  Port=3
  phi_g_in : Inport  Port=4
  Degrees to Radians : simulink_extras/Transformations/Degrees to Radians
  Scope : Scope
      settings: ActiveDisplayYMinimum=-38.976572613455062  ActiveDisplayYMaximum=38.12312470041  DataLoggingVariableName=ScopeData5
  Scope1 : Scope
      settings: ActiveDisplayYMinimum=0.0017996827006821164  ActiveDisplayYMaximum=0.0018001989414186065  DataLoggingVariableName=ScopeData8
  Scope2 : Scope
      settings: ActiveDisplayYMinimum=-0.28077479370927866  ActiveDisplayYMaximum=0.23553260440653867  DataLoggingVariableName=ScopeData6
  Subsystem : Subsystem
  caculateZ1F1 : Subsystem
  caculateZ2 : Subsystem
  deltaChi : Sum  Inputs=-+|
  phiLimit : Saturate  UpperLimit=30/57.3  LowerLimit=-30/57.3
  theta1 : Selector  InputPortWidth=21  IndexOptions=Index vector (dialog)  Indices=15  OutputSizes=[(-2)]
  theta3 : Selector  InputPortWidth=21  IndexOptions=Index vector (dialog)  Indices=14  OutputSizes=[(-2)]
  phi_g_rad : Outport
  wires:
  [Plane_Data] -> theta3/1
  phiLimit/1 -> phi_g_rad/1, Scope2/1
  Chi_g/1 -> Degrees to Radians/1
  theta1/1 -> deltaChi/2
  theta3/1 -> [vGnd], caculateZ1F1/2(vGnd)
  [Plane_Data] -> theta1/1
  caculateZ1F1/2(f1) -> [f1]
  caculateZ1F1/1(z1) -> Scope1/1, [z1]
  deltaChi/1 -> [deltaChi], caculateZ2/1(deltaChi)
  [z1] -> caculateZ2/2(z1)
  caculateZ2/1(z2) -> [z2]
  Degrees to Radians/1 -> deltaChi/1
  [z2] -> Subsystem/1(z2)
  [z1] -> Subsystem/2(z1)
  [f1] -> Subsystem/3(f1)
  [deltaChi] -> Subsystem/4(deltaChi)
  [vGnd] -> Subsystem/5(vGnd)
  phi_g_in/1 -> Subsystem/6(phi_g_in)
  legType/1 -> Subsystem/7(legType)
  Subsystem/1(phiCmd) -> phiLimit/1
  YZ/1 -> Scope/1, caculateZ1F1/1(YZ)

== system AFCSModel/RNP AR Approach Guidance/ndiControl ==
  note: 动态逆控制
  legType : Inport
  Chi_g : Inport  Port=2
  YZ : Inport  Port=3
  phi_g_in : Inport  Port=4
  Constant : Constant  Value=-0.3
  Degrees to Radians : simulink_extras/Transformations/Degrees to Radians
  Gain1 : Gain  Gain=0.035
  Product : Product
  Product1 : Product
  Scope : Scope
      settings: ActiveDisplayYMinimum=-30.880204914689969  ActiveDisplayYMaximum=22.015235326559953
  Sin : Trigonometry
  Sum : Sum  Inputs=|++
  Sum2 : Sum  Inputs=|-+
  Switch : Switch  Criteria=u2 > Threshold  Threshold=0.5  SaturateOnIntegerOverflow=off  InputSameDT=off
  calculatePhi : Subsystem
  phiLimit : Saturate  UpperLimit=30/57.3  LowerLimit=-30/57.3
  theta1 : Selector  InputPortWidth=21  IndexOptions=Index vector (dialog)  Indices=15  OutputSizes=[(-2)]
  theta3 : Selector  InputPortWidth=21  IndexOptions=Index vector (dialog)  Indices=14  OutputSizes=[(-2)]
  phi_g : Outport
  wires:
  legType/1 -> Switch/2
  Switch/1 -> phiLimit/1
  [Plane_Data] -> theta1/1, theta3/1
  phiLimit/1 -> phi_g/1
  YZ/1 -> Scope/1, Gain1/1
  calculatePhi/2(tfPhi) -> Switch/3
  Sum/1 -> calculatePhi/1(vControl)
  theta1/1 -> Sum2/2
  Chi_g/1 -> Degrees to Radians/1
  Sum2/1 -> calculatePhi/2(deltaChi), Sin/1
  theta3/1 -> calculatePhi/3(vGnd), Product1/2
  phi_g_in/1 -> calculatePhi/4(phi_g_in)
  calculatePhi/1(rfPhi) -> Switch/1
  Degrees to Radians/1 -> Sum2/1
  Constant/1 -> Product/1
  Product1/1 -> [derr]
  [derr] -> Product/2
  Sin/1 -> Product1/1
  Product/1 -> Sum/1
  Gain1/1 -> Sum/2

== system AFCSModel/VS_modify/Pitch_modify ==
  note: theta
  theta_g : Inport
  Constant3 : Constant  Value=op.States(3).x(2)
  Gain : Gain  Gain=2.6
  Gain1 : Gain  Gain=2
  Selector : Selector  InputPortWidth=21  IndexOptions=Index vector (dialog)  Indices=8  OutputSizes=1
  Selector1 : Selector  InputPortWidth=21  IndexOptions=Index vector (dialog)  Indices=5  OutputSizes=1
  Sum1 : Sum  Inputs=|++
  Sum2 : Sum  Inputs=|++
  Sum3 : Sum  Inputs=|-+
  delta_e : Outport
  wires:
  Sum1/1 -> delta_e/1
  Selector1/1 -> Gain1/1  "q"
  Sum3/1 -> Gain/1
  Sum2/1 -> Sum3/1
  Constant3/1 -> Sum2/2
  theta_g/1 -> Sum2/1
  Gain/1 -> Sum1/1
  Gain1/1 -> Sum1/2
  [Plane_Data] -> Selector/1, Selector1/1
  Selector/1 -> Sum3/2

== system AFCSModel/Wind_Model/DCM_e2b ==
  euler : Inport
  A11 : Subsystem
  A12 : Subsystem
  A13 : Subsystem
  A21 : Subsystem
  A22 : Subsystem
  A23 : Subsystem
  A31 : Subsystem
  A32 : Subsystem
  A33 : Subsystem
  Create Transformation Matrix : sharedutil/Create 3x3 Matrix  aMode=aMode
      settings: LibrarySourceBlock=aerolibutil/Create 3x3 Matrix
  Demux2 : Demux  Outputs=3
  Mux : Mux  Inputs=6
  sincos : Trigonometry  Operator=sincos
  sincos1 : Trigonometry  Operator=sincos
  sincos2 : Trigonometry  Operator=sincos
  DCM : Outport  PortDimensions=[3,3]  InitialOutput=0
  wires:
  A12/1(A12) -> Create Transformation Matrix/2
  A21/1(A21) -> Create Transformation Matrix/4
  A32/1(A32) -> Create Transformation Matrix/8
  A22/1(A22) -> Create Transformation Matrix/5
  A23/1(A23) -> Create Transformation Matrix/6
  A31/1(A31) -> Create Transformation Matrix/7
  Mux/1 -> A22/1(sin_cos), A23/1(sin_cos), A31/1(sin_cos), A32/1(sin_cos), A33/1(sin_cos), A21/1(sin_cos), A13/1(sin_cos), A12/1(sin_cos), A11/1(sin_cos)
  Create Transformation Matrix/1 -> DCM/1
  A33/1(A33) -> Create Transformation Matrix/9
  A11/1(A11) -> Create Transformation Matrix/1
  A13/1(A13) -> Create Transformation Matrix/3
  Demux2/1 -> sincos/1
  Demux2/2 -> sincos1/1
  Demux2/3 -> sincos2/1
  sincos/1 -> Mux/1
  sincos/2 -> Mux/2
  sincos1/1 -> Mux/3
  sincos1/2 -> Mux/4
  sincos2/1 -> Mux/5
  sincos2/2 -> Mux/6
  euler/1 -> Demux2/1

== system AFCSModel/Plane&Actuator/Actuator/actuator1 ==
  In : Inport
  -24  +24 : Saturate  UpperLimit=150  LowerLimit=-150  LinearizeAsGain=off
  -30  +30 : Saturate  UpperLimit=30  LowerLimit=-30
  Gain1 : Gain  SaturateOnIntegerOverflow=on  OutDataTypeStr=Inherit: Same as input  ParamDataTypeStr=Inherit: Same as input
  Gain2 : Gain  Gain=100  SaturateOnIntegerOverflow=on  OutDataTypeStr=Inherit: Same as input  ParamDataTypeStr=Inherit: Same as input
  Gain3 : Gain  SaturateOnIntegerOverflow=on  OutDataTypeStr=Inherit: Same as input  ParamDataTypeStr=Inherit: Same as input
  Integrator1 : Integrator
  Sum10 : Sum  Inputs=+-  InputSameDT=on  SaturateOnIntegerOverflow=on  OutDataTypeStr=Inherit: Same as first input
  Transfer Fcn : TransferFcn  Denominator=[0.0151 1]
  Out : Outport
  wires:
  Gain2/1 -> -24  +24/1
  Gain3/1 -> Sum10/2
  -24  +24/1 -> Integrator1/1
  -30  +30/1 -> Gain3/1, Gain1/1
  Transfer Fcn/1 -> Out/1
  Integrator1/1 -> -30  +30/1
  In/1 -> Sum10/1
  Sum10/1 -> Gain2/1
  Gain1/1 -> Transfer Fcn/1

== system AFCSModel/Plane&Actuator/Actuator/actuator3 ==
  In : Inport
  -24  +24 : Saturate  UpperLimit=150  LowerLimit=-150  LinearizeAsGain=off
  -30  +30 : Saturate  UpperLimit=30  LowerLimit=-30
  Gain1 : Gain  SaturateOnIntegerOverflow=on  OutDataTypeStr=Inherit: Same as input  ParamDataTypeStr=Inherit: Same as input
  Gain2 : Gain  Gain=100  SaturateOnIntegerOverflow=on  OutDataTypeStr=Inherit: Same as input  ParamDataTypeStr=Inherit: Same as input
  Gain3 : Gain  SaturateOnIntegerOverflow=on  OutDataTypeStr=Inherit: Same as input  ParamDataTypeStr=Inherit: Same as input
  Integrator1 : Integrator
  Sum10 : Sum  Inputs=+-  InputSameDT=on  SaturateOnIntegerOverflow=on  OutDataTypeStr=Inherit: Same as first input
  Transfer Fcn : TransferFcn  Denominator=[0.0151 1]
  Out : Outport
  wires:
  Gain1/1 -> Transfer Fcn/1
  Sum10/1 -> Gain2/1
  In/1 -> Sum10/1
  Integrator1/1 -> -30  +30/1
  Transfer Fcn/1 -> Out/1
  -30  +30/1 -> Gain1/1, Gain3/1
  -24  +24/1 -> Integrator1/1
  Gain3/1 -> Sum10/2
  Gain2/1 -> -24  +24/1

== system AFCSModel/Plane&Actuator/Actuator/actuator5 ==
  In : Inport
  -24  +24 : Saturate  UpperLimit=150  LowerLimit=-150  LinearizeAsGain=off
  -30  +30 : Saturate  UpperLimit=30  LowerLimit=-30
  Gain1 : Gain  SaturateOnIntegerOverflow=on  OutDataTypeStr=Inherit: Same as input  ParamDataTypeStr=Inherit: Same as input
  Gain2 : Gain  Gain=100  SaturateOnIntegerOverflow=on  OutDataTypeStr=Inherit: Same as input  ParamDataTypeStr=Inherit: Same as input
  Gain3 : Gain  SaturateOnIntegerOverflow=on  OutDataTypeStr=Inherit: Same as input  ParamDataTypeStr=Inherit: Same as input
  Integrator1 : Integrator
  Sum10 : Sum  Inputs=+-  InputSameDT=on  SaturateOnIntegerOverflow=on  OutDataTypeStr=Inherit: Same as first input
  Transfer Fcn : TransferFcn  Denominator=[0.0151 1]
  Out : Outport
  wires:
  Gain1/1 -> Transfer Fcn/1
  Sum10/1 -> Gain2/1
  In/1 -> Sum10/1
  Integrator1/1 -> -30  +30/1
  Transfer Fcn/1 -> Out/1
  -30  +30/1 -> Gain1/1, Gain3/1
  -24  +24/1 -> Integrator1/1
  Gain3/1 -> Sum10/2
  Gain2/1 -> -24  +24/1

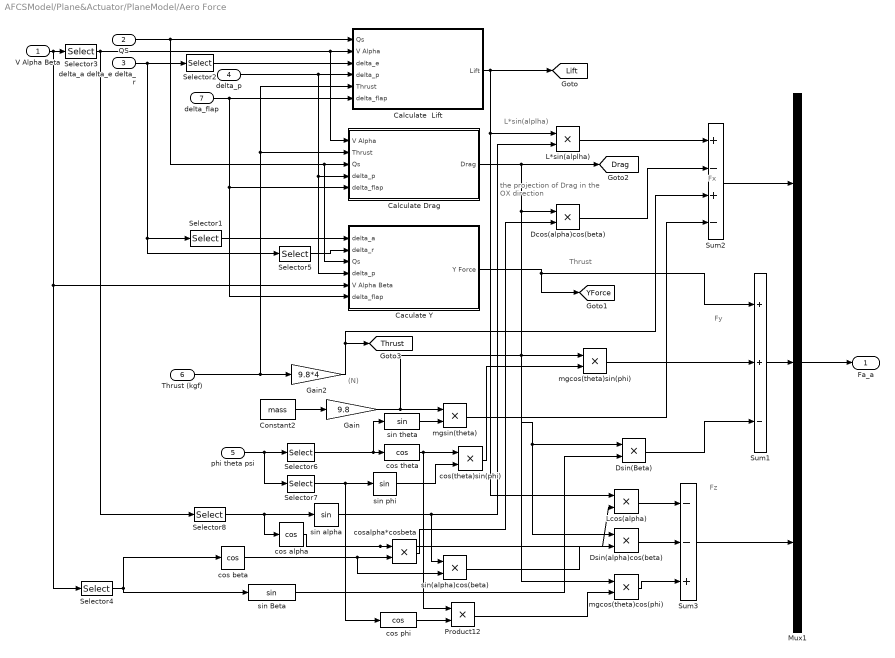
== system AFCSModel/Plane&Actuator/PlaneModel/Aero Force ==
  note: Fx
  note: L*sin(alplha)
  note: the projection of Drag
      | in the OX direction
  note: Fy
  note: Fz
  note: Thrust
  note: (N)
  V Alpha Beta : Inport
  QS : Inport  Port=2
  delta_a delta_e delta_r : Inport  Port=3
  delta_p : Inport  Port=4
  phi theta psi : Inport  Port=5
  Thrust (kgf) : Inport  Port=6
  delta_flap : Inport  Port=7
  Caculate Y : Subsystem
  Calculate  Lift : Subsystem
  Calculate Drag : Subsystem
  Constant2 : Constant  Value=mass  OutDataTypeStr=Inherit: Inherit via back propagation
  Dcos(alpha)cos(beta) : Product  RndMeth=Zero
  Dsin(Beta) : Product  RndMeth=Zero
  Dsin(alpha)cos(beta) : Product  RndMeth=Zero
  Gain : Gain  Gain=9.8
  Gain2 : Gain  Gain=9.8*4
  L*sin(alplha) : Product  RndMeth=Zero
  Lcos(alpha) : Product  RndMeth=Zero
  Mux1 : Mux  Inputs=3
  Product12 : Product  RndMeth=Zero
  Selector1 : Selector  InputPortWidth=3  IndexOptions=Index vector (dialog)  Indices=[1]  OutputSizes=[(-2)]
  Selector2 : Selector  InputPortWidth=3  IndexOptions=Index vector (dialog)  Indices=[2]  OutputSizes=[(-2)]
  Selector3 : Selector  InputPortWidth=3  IndexOptions=Index vector (dialog)  Indices=[1 2]  OutputSizes=[(-2)]
  Selector4 : Selector  InputPortWidth=3  IndexOptions=Index vector (dialog)  Indices=[3]  OutputSizes=[(-2)]
  Selector5 : Selector  InputPortWidth=3  IndexOptions=Index vector (dialog)  Indices=[3]  OutputSizes=[(-2)]
  Selector6 : Selector  InputPortWidth=3  IndexOptions=Index vector (dialog)  Indices=[2]  OutputSizes=[(-2)]
  Selector7 : Selector  InputPortWidth=3  IndexOptions=Index vector (dialog)  Indices=[1]  OutputSizes=[(-2)]
  Selector8 : Selector  InputPortWidth=2  IndexOptions=Index vector (dialog)  Indices=[2]  OutputSizes=[(-2)]
  Sum1 : Sum  Inputs=++-
  Sum2 : Sum  Inputs=+-+-
  Sum3 : Sum  Inputs=--+
  cos alpha : Trigonometry  Operator=cos
  cos beta : Trigonometry  Operator=cos
  cos phi : Trigonometry  Operator=cos
  cos theta : Trigonometry  Operator=cos
  cos(theta)sin(phi) : Product  RndMeth=Zero
  cosalpha*cosbeta : Product  RndMeth=Zero
  mgcos(theta)cos(phi) : Product  RndMeth=Zero
  mgcos(theta)sin(phi) : Product  RndMeth=Zero
  mgsin(theta) : Product  RndMeth=Zero
  sin Beta : Trigonometry
  sin alpha : Trigonometry
  sin phi : Trigonometry
  sin theta : Trigonometry
  sin(alpha)cos(beta) : Product  RndMeth=Zero
  Fa_a : Outport
  tag scope: Drag=global, Lift=global, Thrust=global, YForce=global
  wires:
  delta_a delta_e delta_r/1 -> Selector2/1, Selector5/1, Selector1/1
  Selector3/1 -> Selector8/1, Calculate  Lift/2(" V Alpha"), Calculate Drag/1(" V Alpha")
  Mux1/1 -> Fa_a/1
  Sum2/1 -> Mux1/1
  delta_p/1 -> Calculate Drag/4(delta_p), Caculate Y/4(delta_p), Calculate  Lift/4(delta_p)
  QS/1 -> Calculate  Lift/1(Qs), Calculate Drag/3(Qs), Caculate Y/3(Qs)
  Selector2/1 -> Calculate  Lift/3(delta_e)
  V Alpha Beta/1 -> Selector4/1, Caculate Y/5(" V Alpha Beta"), Selector3/1
  Calculate  Lift/1(Lift) -> Lcos(alpha)/1, L*sin(alplha)/1, [Lift]
  L*sin(alplha)/1 -> Sum2/1
  Calculate Drag/1(Drag) -> [Drag], Dsin(Beta)/1, Dsin(alpha)cos(beta)/1, Dcos(alpha)cos(beta)/1
  cosalpha*cosbeta/1 -> Dcos(alpha)cos(beta)/2
  Dcos(alpha)cos(beta)/1 -> Sum2/2
  Thrust (kgf)/1 -> Gain2/1, Calculate  Lift/5(Thrust), Calculate Drag/2(Thrust)
  phi theta psi/1 -> Selector6/1, Selector7/1
  mgsin(theta)/1 -> Sum2/4
  Caculate Y/1(Y Force) -> [YForce], Sum1/1
  Sum1/1 -> Mux1/2
  mgcos(theta)sin(phi)/1 -> Sum1/2
  Dsin(Beta)/1 -> Sum1/3
  Sum3/1 -> Mux1/3
  Lcos(alpha)/1 -> Sum3/1
  Dsin(alpha)cos(beta)/1 -> Sum3/2
  mgcos(theta)cos(phi)/1 -> Sum3/3
  Selector1/1 -> Caculate Y/1(delta_a)
  Selector5/1 -> Caculate Y/2(delta_r)
  Gain2/1 -> [Thrust], Sum2/3
  Selector8/1 -> sin alpha/1, cos alpha/1
  Product12/1 -> mgcos(theta)cos(phi)/2
  cos phi/1 -> Product12/2
  sin(alpha)cos(beta)/1 -> Dsin(alpha)cos(beta)/2
  sin Beta/1 -> Dsin(Beta)/2
  cos(theta)sin(phi)/1 -> mgcos(theta)sin(phi)/2
  cos theta/1 -> cos(theta)sin(phi)/1, Product12/1
  sin phi/1 -> cos(theta)sin(phi)/2
  Selector7/1 -> sin phi/1, cos phi/1
  cos beta/1 -> cosalpha*cosbeta/2, sin(alpha)cos(beta)/2
  cos alpha/1 -> cosalpha*cosbeta/1, Lcos(alpha)/2
  sin alpha/1 -> sin(alpha)cos(beta)/1, L*sin(alplha)/2
  sin theta/1 -> mgsin(theta)/2
  Selector6/1 -> sin theta/1, cos theta/1
  Gain/1 -> mgsin(theta)/1, mgcos(theta)cos(phi)/1, mgcos(theta)sin(phi)/1
  Constant2/1 -> Gain/1
  Selector4/1 -> cos beta/1, sin Beta/1
  delta_flap/1 -> Calculate  Lift/6(delta_flap), Calculate Drag/5(delta_flap), Caculate Y/6(delta_flap)
